simulink model "lab1_1"  (R2022a)
settings: Solver=ode4  StartTime=0.0  StopTime=10.0  FixedStep=0.001  RelTol=1e-3
settings Model: Creator=Paulo  LastModifiedBy=Paulo
settings SolverCC: AutoInsertRateTranBlk=on

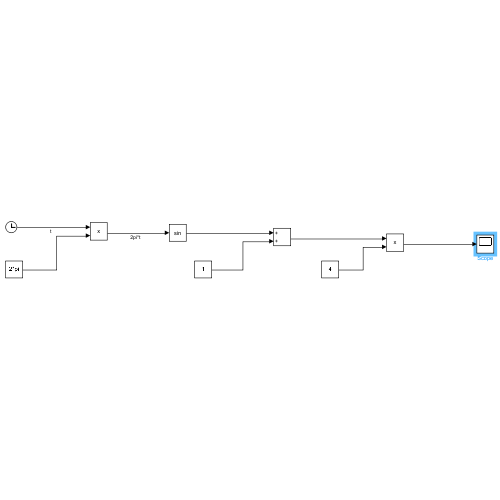
[thumbnail: Simulink's stored preview of the top-level diagram]
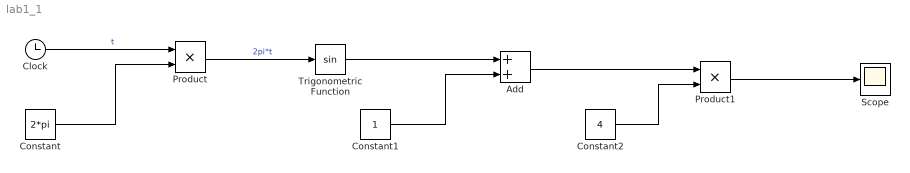
== system lab1_1 ==
  Add : Sum
  Clock : Clock
  Constant : Constant  Value=2*pi
  Constant1 : Constant
  Constant2 : Constant  Value=4
  Product : Product
  Product1 : Product
  Scope : Scope
  Trigonometric Function : Trigonometry
  wires:
  Clock/1 -> Product/1  "t"
  Constant/1 -> Product/2
  Product/1 -> Trigonometric Function/1  "2pi*t"
  Trigonometric Function/1 -> Add/1
  Constant1/1 -> Add/2
  Add/1 -> Product1/1
  Constant2/1 -> Product1/2
  Product1/1 -> Scope/1
